simulink model "PMSM_RFOC"  (R2020a)
settings: Solver=VariableStepAuto  StartTime=0.0  StopTime=10  RelTol=1e-3
settings Model: Creator=alfan  LastModifiedBy=alfan

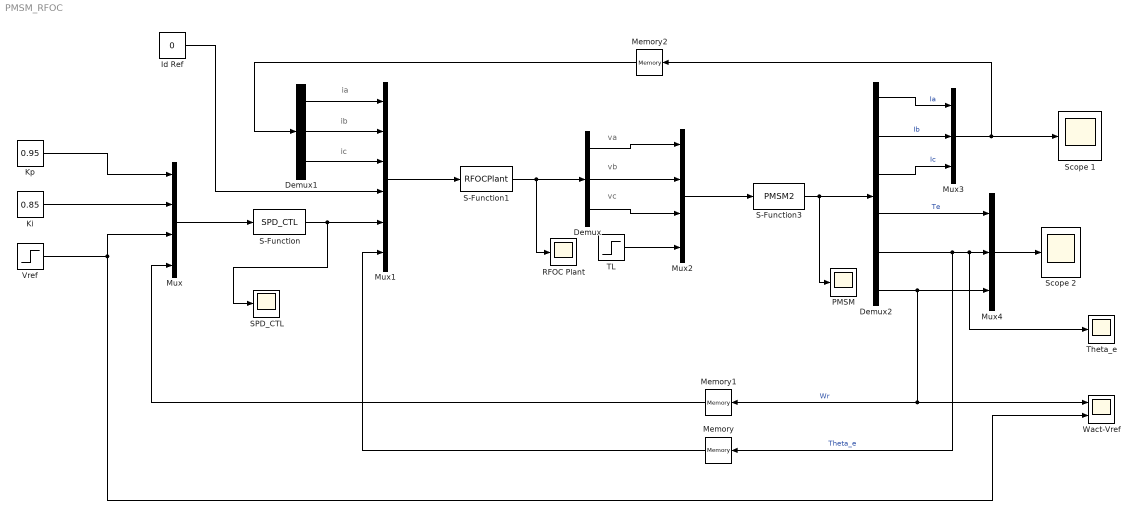
== system PMSM_RFOC ==
  note: ia
  note: ib
  note: ic
  note: va
  note: vb
  note: vc
  Demux : Demux  Outputs=3
  Demux1 : Demux  Outputs=3
  Demux2 : Demux  Outputs=6
  Id Ref : Constant  Value=0
  Ki : Constant  Value=0.85
  Kp : Constant  Value=0.95
  Memory : Memory  InheritSampleTime=on
  Memory1 : Memory
  Memory2 : Memory
  Mux : Mux
  Mux1 : Mux  Inputs=6
  Mux2 : Mux
  Mux3 : Mux  Inputs=3
  Mux4 : Mux  Inputs=3
  PMSM : Scope
  RFOC Plant : Scope
  S-Function : S-Function  FunctionName=SPD_CTL  SFunctionDeploymentMode=off  EnableBusSupport=off
  S-Function1 : S-Function  FunctionName=RFOCPlant  SFunctionDeploymentMode=off  EnableBusSupport=off
  S-Function3 : S-Function  FunctionName=PMSM2  SFunctionDeploymentMode=off  EnableBusSupport=off
  SPD_CTL : Scope
  Scope 1 : Scope
  Scope 2 : Scope
  TL : Step  After=3  SampleTime=0
  Theta_e : Scope
  Vref : Step  Time=3  After=10  SampleTime=0
  Wact-Vref : Scope  NumInputPorts=2
  wires:
  Kp/1 -> Mux/1
  Ki/1 -> Mux/2
  Vref/1 -> Wact-Vref/2, Mux/3
  Mux/1 -> S-Function/1
  S-Function/1 -> SPD_CTL/1, Mux1/5
  Mux1/1 -> S-Function1/1
  S-Function1/1 -> RFOC Plant/1, Demux/1
  TL/1 -> Mux2/4
  Demux/3 -> Mux2/3
  Demux/2 -> Mux2/2
  Demux/1 -> Mux2/1
  Demux1/1 -> Mux1/1
  Demux1/2 -> Mux1/2
  Demux1/3 -> Mux1/3
  Mux2/1 -> S-Function3/1
  S-Function3/1 -> PMSM/1, Demux2/1
  Demux2/5 -> Memory/1, Theta_e/1, Mux4/2  "Theta_e"
  Memory1/1 -> Mux/4
  Demux2/1 -> Mux3/1  "Ia"
  Demux2/2 -> Mux3/2  "Ib"
  Demux2/3 -> Mux3/3  "Ic"
  Mux3/1 -> Memory2/1, Scope 1/1
  Memory2/1 -> Demux1/1
  Demux2/4 -> Mux4/1  "Te"
  Demux2/6 -> Wact-Vref/1, Memory1/1, Mux4/3  "Wr"
  Mux4/1 -> Scope 2/1
  Memory/1 -> Mux1/6
  Id Ref/1 -> Mux1/4
